simulink model "SIM_linear"  (R2023a)
settings: Solver=VariableStepAuto  StartTime=0.0  StopTime=20  MaxStep=1e-5  RelTol=1e-3
values from neighbouring files (symbols this model uses):
  A = [0 0 0 1 0 0 ... (first row only)    [param.m]
  B = [0; 0; 0; B_part_num(1); B_part_num(2); B_part_num(3)]    [param.m]
  C = eye(6)    [param.m]
  Kr = sqrt(Q(1, 1)/R)    [param.m]
  theta1_rad = theta1_deg * pi / 180    (= 0.0174532925199)    [param.m]
  theta2_rad = theta2_deg * pi / 180    (= -0.0174532925199)    [param.m]
undefined symbols (not defined in the file or in its folder): K
settings Model: SimulationMode=accelerator  Creator=edzel  LastModifiedBy=edzel

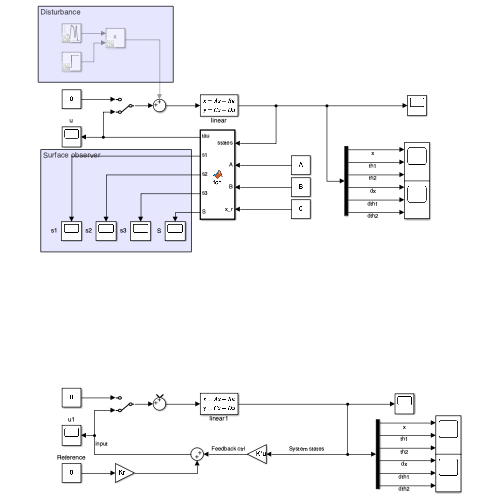
[thumbnail: Simulink's stored preview of the top-level diagram]
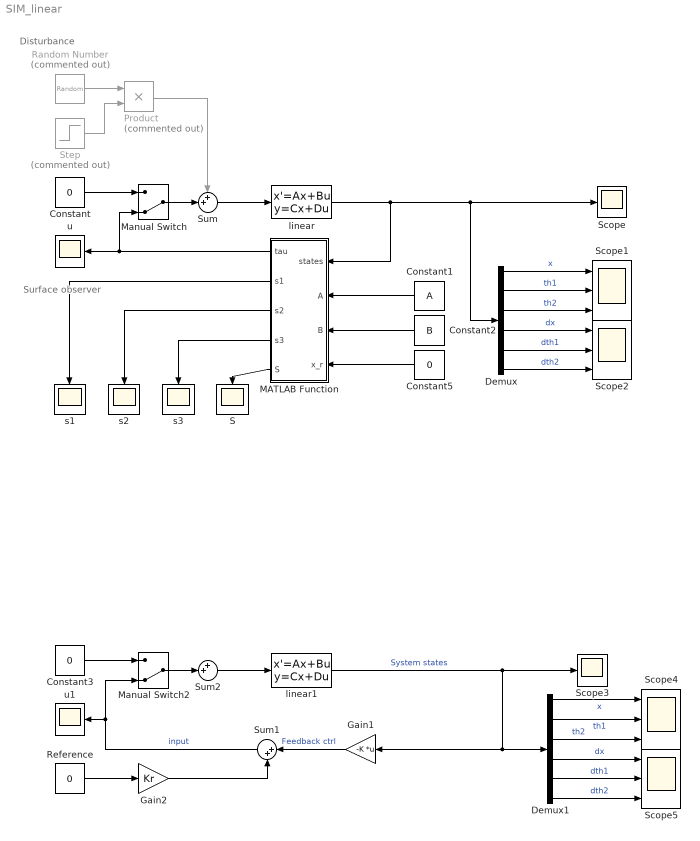
== system SIM_linear ==
  note: Disturbance
  note: Surface observer
  Constant : Constant  Value=0
  Constant1 : Constant  Value=A
  Constant2 : Constant  Value=B
  Constant3 : Constant  Value=0
  Constant5 : Constant  Value=0
  Demux : Demux  Outputs=6
  Demux1 : Demux  Outputs=6
  Gain1 : Gain  Gain=-K  Multiplication=Matrix(K*u)
  Gain2 : Gain  Gain=Kr
  MATLAB Function : MATLAB Function  TreatAsAtomicUnit=on
  Manual Switch : ManualSwitch  CurrentSetting=0
  Manual Switch2 : ManualSwitch  CurrentSetting=0
  Product : Product  Commented=on
  Random Number : RandomNumber  Commented=on  SampleTime=0.1
  Reference : Constant  Value=0
  S : Scope
  Scope : Scope
  Scope{1..2,4..5} (4 alike) : Scope  NumInputPorts=3
  Scope3 : Scope
  Step : Step  Commented=on  SampleTime=0
  Sum : Sum  Inputs=++|
  Sum1 : Sum  Inputs=|++
  Sum2 : Sum  Inputs=++|
  linear : StateSpace  A=A  B=B  C=C  D=zeros(6, 1)  InitialCondition=[0; theta1_rad; theta2_rad; 0; 0; 0]
  linear1 : StateSpace  A=A  B=B  C=C  D=zeros(6, 1)  InitialCondition=[0; theta1_rad; theta2_rad; 0; 0; 0]
  s1 : Scope
  s2 : Scope
  s3 : Scope
  u : Scope
  u1 : Scope
  wires:
  Constant/1 -> Manual Switch/1
  linear/1 -> MATLAB Function/1(states), Scope/1, Demux/1
  Constant1/1 -> MATLAB Function/2(A)
  Constant2/1 -> MATLAB Function/3(B)
  Constant5/1 -> MATLAB Function/4(x_r)
  Demux/1 -> Scope1/1  "x"
  Demux/2 -> Scope1/2  "th1"
  Demux/3 -> Scope1/3  "th2"
  Demux/4 -> Scope2/1  "dx"
  Demux/5 -> Scope2/2  "dth1"
  Demux/6 -> Scope2/3  "dth2"
  MATLAB Function/2(s1) -> s1/1
  MATLAB Function/3(s2) -> s2/1
  MATLAB Function/4(s3) -> s3/1
  MATLAB Function/5(S) -> S/1
  MATLAB Function/1(tau) -> Manual Switch/2, u/1
  Constant3/1 -> Manual Switch2/1
  Demux1/6 -> Scope5/3  "dth2"
  Reference/1 -> Gain2/1
  Demux1/4 -> Scope5/1  "dx"
  Demux1/1 -> Scope4/1  "x"
  Demux1/5 -> Scope5/2  "dth1"
  Demux1/2 -> Scope4/2  "th1"
  Demux1/3 -> Scope4/3  "th2"
  Sum1/1 -> u1/1, Manual Switch2/2  "input"
  linear1/1 -> Scope3/1, Gain1/1, Demux1/1  "System states"
  Gain2/1 -> Sum1/2
  Gain1/1 -> Sum1/1  "Feedback ctrl"
  Sum/1 -> linear/1
  Manual Switch/1 -> Sum/2
  Random Number/1 -> Product/1
  Step/1 -> Product/2
  Product/1 -> Sum/1
  Sum2/1 -> linear1/1
  Manual Switch2/1 -> Sum2/2

== matlab function SIM_linear/MATLAB Function ==
  data: states input; tau output; A input; B input; x_r input; s1 output; s2 output; s3 output; S output
function [tau, s1, s2, s3, S] = fcn(states, A, B, x_r)

c1 = 2;       % 2
c2 = 5;         % 5
c3 = 1.3;       % 1.6 - 1.7？

alpha = 1.5;    % 1.5
beta =  4.4;     % 4.4
gamma = 2.7;    % 2.7

eta = 0.005;    % 0.005
k = 10;         % 20

x = states(1);
th1 = states(2);
th2 = states(3);

dx = states(4);
dth1 = states(5);
dth2 = states(6);

s1 = c1 * th1 + dth1;
s2 = c2 * th2 + dth2;
s3 = c3 * (x-x_r) + dx;

b1 = B(5, 1);
b2 = B(6, 1);
b3 = B(4, 1);

S = alpha * s1 + beta * s2 + gamma * s3;

% ueq1 = -(c1*dth1 + A(5,2)*th1 + A(5,3)*th2)/b1;
b1ueq1 = -(c1*dth1 + A(5,2)*th1 + A(5,3)*th2);

% ueq2 = -(c2*dth2 + A(6,2)*th1 + A(6,3)*th2)/b2;
b2ueq2 = -(c2*dth2 + A(6,2)*th1 + A(6,3)*th2);

% ueq3 = -(c3*dx + A(4,2)*th1 + A(4,3)*th2)/b3;
b3ueq3 = -(c3*dx + A(4,2)*th1 + A(4,3)*th2);

den = alpha * b1 + beta * b2 + gamma * b3;

u = (alpha*b1ueq1 + beta*b2ueq2 + gamma*b3ueq3 - eta*sign(S) -k*S) / den;

tau = u;


% Current advantage for SMC over LQR: better response at a cost of larger 
% angle change, but with smaller input.
% Not ideal for any desired destination.
% Good comparison at x_ref = 0.
